simulink model "RST_Simulink_1ªordem"  (R2018b)
settings: Solver=VariableStepAuto  StartTime=0.0  StopTime=10.0  RelTol=1e-3
values from neighbouring files (symbols this model uses):
  A = den    [cod_teste_RST_2.m]
  B = num    (= 1)    [cod_teste_RST_2.m]
  R = X(1)    [cod_teste_RST_1.m]    (also in cod_teste_RST_2.m = [1 X(1)])
  S = X(2:end)    [cod_teste_RST_1.m]    (also in cod_teste_RST_2.m = [X(3) X(2)])
  T = sum(PMF)/sum(B)    [cod_teste_RST_1.m]    (also in cod_teste_RST_2.m = sum(Am)/sum(B))
settings Model: Creator=tarci  LastModifiedBy=tarci

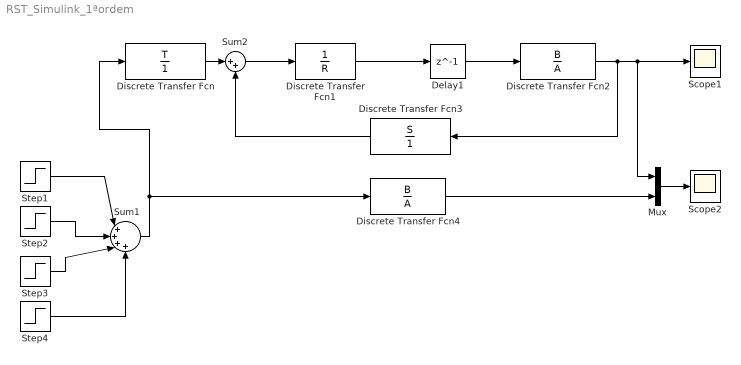
== system RST_Simulink_1ªordem ==
  Delay1 : Delay  DelayLength=1  InitialCondition=0
  Discrete Transfer Fcn : DiscreteTransferFcn  Numerator=T  Denominator=[1]
  Discrete Transfer Fcn1 : DiscreteTransferFcn  Denominator=R
  Discrete Transfer Fcn2 : DiscreteTransferFcn  Numerator=B  Denominator=A
  Discrete Transfer Fcn3 : DiscreteTransferFcn  Numerator=S  Denominator=[1]
  Discrete Transfer Fcn4 : DiscreteTransferFcn  Numerator=B  Denominator=A
  Mux : Mux  Inputs=2
  Scope1 : Scope
  Scope2 : Scope
  Step1 : Step  Time=0  SampleTime=0
  Step2 : Step  Time=10  After=3  SampleTime=0
  Step3 : Step  Time=15  After=2  SampleTime=0
  Step4 : Step  Time=20  SampleTime=0
  Sum1 : Sum  Inputs=|++++
  Sum2 : Sum  Inputs=|++
  wires:
  Discrete Transfer Fcn1/1 -> Delay1/1
  Discrete Transfer Fcn/1 -> Sum2/1
  Delay1/1 -> Discrete Transfer Fcn2/1
  Sum2/1 -> Discrete Transfer Fcn1/1
  Discrete Transfer Fcn3/1 -> Sum2/2
  Discrete Transfer Fcn2/1 -> Mux/1, Scope1/1, Discrete Transfer Fcn3/1
  Discrete Transfer Fcn4/1 -> Mux/2
  Mux/1 -> Scope2/1
  Step1/1 -> Sum1/1
  Step2/1 -> Sum1/2
  Step3/1 -> Sum1/3
  Step4/1 -> Sum1/4
  Sum1/1 -> Discrete Transfer Fcn4/1, Discrete Transfer Fcn/1
